simulink model "TST_Fans_trq"  (R2016b)
settings: Solver=FixedStepDiscrete  StartTime=0.0  StopTime=simTime  FixedStep=sampleTime  RelTol=1e-3
values from neighbouring files (symbols this model uses):
  testCase = 1    [initTST_Fans_trq_001.m]    (also in initTST_Fans_trq_002.m = 2)
libraries: simulink x7, UnitTest_Lib x4
settings Model: Creator=zhengjinyan  LastModifiedBy=zhengjinyan
settings DebuggingCC: SignalRangeChecking=error

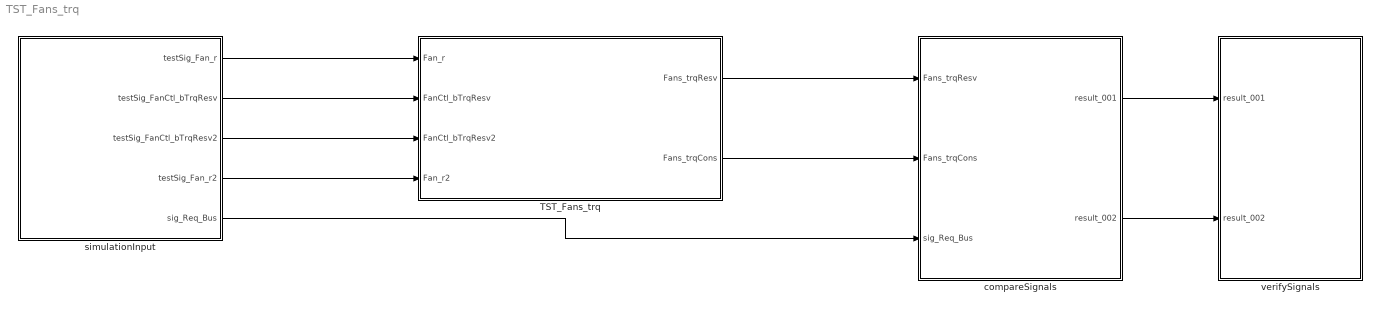
== system TST_Fans_trq ==
  TST_Fans_trq : Subsystem
  compareSignals : Subsystem
  simulationInput : Subsystem
  verifySignals : Subsystem
  wires:
  simulationInput/1(testSig_Fan_r) -> TST_Fans_trq/1(Fan_r)
  simulationInput/2(testSig_FanCtl_bTrqResv) -> TST_Fans_trq/2(FanCtl_bTrqResv)
  simulationInput/3(testSig_FanCtl_bTrqResv2) -> TST_Fans_trq/3(FanCtl_bTrqResv2)
  simulationInput/4(testSig_Fan_r2) -> TST_Fans_trq/4(Fan_r2)
  TST_Fans_trq/1(Fans_trqResv) -> compareSignals/1(Fans_trqResv)
  TST_Fans_trq/2(Fans_trqCons) -> compareSignals/2(Fans_trqCons)
  simulationInput/5(sig_Req_Bus) -> compareSignals/3(sig_Req_Bus)
  compareSignals/1(result_001) -> verifySignals/1(result_001)
  compareSignals/2(result_002) -> verifySignals/2(result_002)

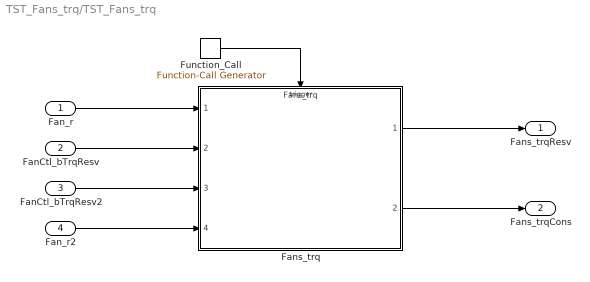
== system TST_Fans_trq/TST_Fans_trq ==
  Fan_r : Inport
  FanCtl_bTrqResv : Inport  Port=2
  FanCtl_bTrqResv2 : Inport  Port=3
  Fan_r2 : Inport  Port=4
  Fans_trq : ModelReference  ModelNameDialog=Fans_trq  SimulationMode=Normal  ModelReferenceVersion=1.16  TriggerPortName=function  TriggerPortTriggerType=function-call  TriggerPortStatesWhenEnabling=held
  Function_Call : simulink/Ports & Subsystems/Function-Call Generator  sample_time=sampleTime  numberOfIterations=1
  Fans_trqResv : Outport
  Fans_trqCons : Outport  Port=2
  wires:
  Function_Call/1 -> Fans_trq/Trigger
  Fan_r/1 -> Fans_trq/1
  FanCtl_bTrqResv/1 -> Fans_trq/2
  FanCtl_bTrqResv2/1 -> Fans_trq/3
  Fan_r2/1 -> Fans_trq/4
  Fans_trq/1 -> Fans_trqResv/1
  Fans_trq/2 -> Fans_trqCons/1

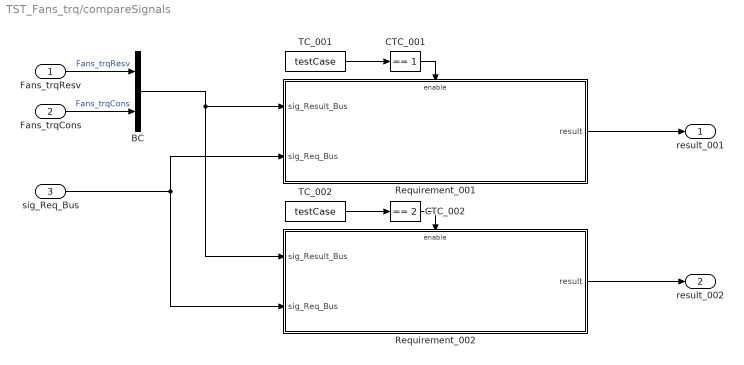
== system TST_Fans_trq/compareSignals ==
  Fans_trqResv : Inport
  Fans_trqCons : Inport  Port=2
  sig_Req_Bus : Inport  Port=3
  BC : BusCreator  Inputs=2
  CTC_001 : simulink/Logic and Bit Operations/Compare To Constant  relop===  const=1  OutDataTypeStr=boolean
  CTC_002 : simulink/Logic and Bit Operations/Compare To Constant  relop===  const=2  OutDataTypeStr=boolean
  Requirement_001 : Subsystem
  Requirement_002 : Subsystem
  TC_001 : Constant  Value=testCase
  TC_002 : Constant  Value=testCase
  result_001 : Outport
  result_002 : Outport  Port=2
  wires:
  Fans_trqResv/1 -> BC/1  "Fans_trqResv"
  Fans_trqCons/1 -> BC/2  "Fans_trqCons"
  TC_001/1 -> CTC_001/1
  CTC_001/1 -> Requirement_001/Enable
  sig_Req_Bus/1 -> Requirement_001/2(sig_Req_Bus), Requirement_002/2(sig_Req_Bus)
  BC/1 -> Requirement_001/1(sig_Result_Bus), Requirement_002/1(sig_Result_Bus)
  Requirement_001/1(result) -> result_001/1
  TC_002/1 -> CTC_002/1
  CTC_002/1 -> Requirement_002/Enable
  Requirement_002/1(result) -> result_002/1

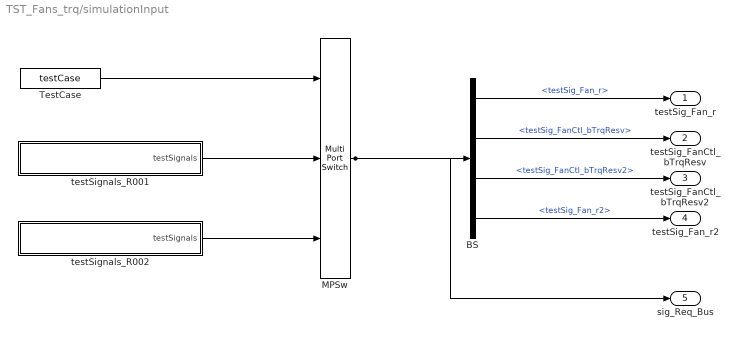
== system TST_Fans_trq/simulationInput ==
  BS : BusSelector  OutputSignals=testSig_Fan_r,testSig_FanCtl_bTrqResv,testSig_FanCtl_bTrqResv2,testSig_Fan_r2
  MPSw : MultiPortSwitch  Inputs=2  SaturateOnIntegerOverflow=on  InputSameDT=on
  TestCase : Constant  Value=testCase
  testSignals_R001 : Subsystem
  testSignals_R002 : Subsystem
  testSig_Fan_r : Outport
  testSig_FanCtl_bTrqResv : Outport  Port=2
  testSig_FanCtl_bTrqResv2 : Outport  Port=3
  testSig_Fan_r2 : Outport  Port=4
  sig_Req_Bus : Outport  Port=5
  wires:
  BS/1 -> testSig_Fan_r/1  "<testSig_Fan_r>"
  BS/2 -> testSig_FanCtl_bTrqResv/1  "<testSig_FanCtl_bTrqResv>"
  BS/3 -> testSig_FanCtl_bTrqResv2/1  "<testSig_FanCtl_bTrqResv2>"
  BS/4 -> testSig_Fan_r2/1  "<testSig_Fan_r2>"
  MPSw/1 -> BS/1, sig_Req_Bus/1
  TestCase/1 -> MPSw/1
  testSignals_R001/1(testSignals) -> MPSw/2
  testSignals_R002/1(testSignals) -> MPSw/3

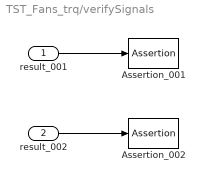
== system TST_Fans_trq/verifySignals ==
  result_001 : Inport
  result_002 : Inport  Port=2
  Assertion_001 : Assertion  Enabled=off
  Assertion_002 : Assertion  Enabled=off
  wires:
  result_001/1 -> Assertion_001/1
  result_002/1 -> Assertion_002/1

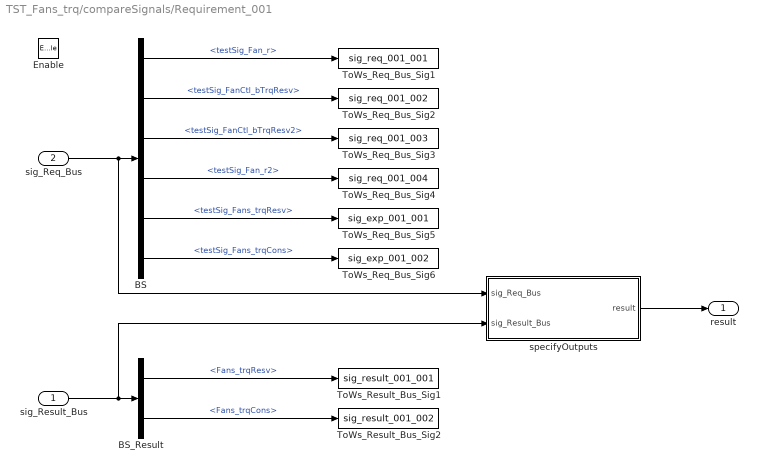
== system TST_Fans_trq/compareSignals/Requirement_001 ==
  sig_Result_Bus : Inport
  sig_Req_Bus : Inport  Port=2
  Enable : EnablePort
  BS : BusSelector  OutputSignals=testSig_Fan_r,testSig_FanCtl_bTrqResv,testSig_FanCtl_bTrqResv2,testSig_Fan_r2,testSig_Fans_trqResv,testSig_Fans_trqCons
  BS_Result : BusSelector  OutputSignals=Fans_trqResv,Fans_trqCons
  ToWs_Req_Bus_Sig1 : ToWorkspace  VariableName=sig_req_001_001  SaveFormat=Structure With Time
  ToWs_Req_Bus_Sig2 : ToWorkspace  VariableName=sig_req_001_002  SaveFormat=Structure With Time
  ToWs_Req_Bus_Sig3 : ToWorkspace  VariableName=sig_req_001_003  SaveFormat=Structure With Time
  ToWs_Req_Bus_Sig4 : ToWorkspace  VariableName=sig_req_001_004  SaveFormat=Structure With Time
  ToWs_Req_Bus_Sig5 : ToWorkspace  VariableName=sig_exp_001_001  SaveFormat=Structure With Time
  ToWs_Req_Bus_Sig6 : ToWorkspace  VariableName=sig_exp_001_002  SaveFormat=Structure With Time
  ToWs_Result_Bus_Sig1 : ToWorkspace  VariableName=sig_result_001_001  SaveFormat=Structure With Time
  ToWs_Result_Bus_Sig2 : ToWorkspace  VariableName=sig_result_001_002  SaveFormat=Structure With Time
  specifyOutputs : Subsystem
  result : Outport
  wires:
  sig_Req_Bus/1 -> BS/1, specifyOutputs/1(sig_Req_Bus)
  BS/1 -> ToWs_Req_Bus_Sig1/1  "<testSig_Fan_r>"
  BS/2 -> ToWs_Req_Bus_Sig2/1  "<testSig_FanCtl_bTrqResv>"
  BS/3 -> ToWs_Req_Bus_Sig3/1  "<testSig_FanCtl_bTrqResv2>"
  BS/4 -> ToWs_Req_Bus_Sig4/1  "<testSig_Fan_r2>"
  BS/5 -> ToWs_Req_Bus_Sig5/1  "<testSig_Fans_trqResv>"
  BS/6 -> ToWs_Req_Bus_Sig6/1  "<testSig_Fans_trqCons>"
  sig_Result_Bus/1 -> BS_Result/1, specifyOutputs/2(sig_Result_Bus)
  BS_Result/1 -> ToWs_Result_Bus_Sig1/1  "<Fans_trqResv>"
  BS_Result/2 -> ToWs_Result_Bus_Sig2/1  "<Fans_trqCons>"
  specifyOutputs/1(result) -> result/1

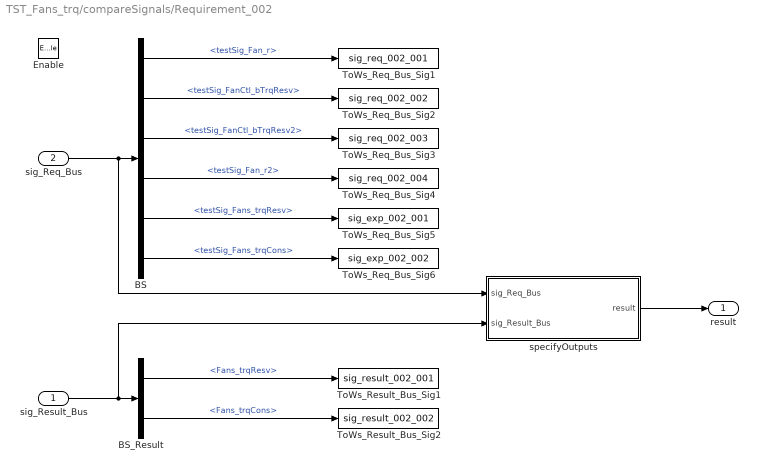
== system TST_Fans_trq/compareSignals/Requirement_002 ==
  sig_Result_Bus : Inport
  sig_Req_Bus : Inport  Port=2
  Enable : EnablePort
  BS : BusSelector  OutputSignals=testSig_Fan_r,testSig_FanCtl_bTrqResv,testSig_FanCtl_bTrqResv2,testSig_Fan_r2,testSig_Fans_trqResv,testSig_Fans_trqCons
  BS_Result : BusSelector  OutputSignals=Fans_trqResv,Fans_trqCons
  ToWs_Req_Bus_Sig1 : ToWorkspace  VariableName=sig_req_002_001  SaveFormat=Structure With Time
  ToWs_Req_Bus_Sig2 : ToWorkspace  VariableName=sig_req_002_002  SaveFormat=Structure With Time
  ToWs_Req_Bus_Sig3 : ToWorkspace  VariableName=sig_req_002_003  SaveFormat=Structure With Time
  ToWs_Req_Bus_Sig4 : ToWorkspace  VariableName=sig_req_002_004  SaveFormat=Structure With Time
  ToWs_Req_Bus_Sig5 : ToWorkspace  VariableName=sig_exp_002_001  SaveFormat=Structure With Time
  ToWs_Req_Bus_Sig6 : ToWorkspace  VariableName=sig_exp_002_002  SaveFormat=Structure With Time
  ToWs_Result_Bus_Sig1 : ToWorkspace  VariableName=sig_result_002_001  SaveFormat=Structure With Time
  ToWs_Result_Bus_Sig2 : ToWorkspace  VariableName=sig_result_002_002  SaveFormat=Structure With Time
  specifyOutputs : Subsystem
  result : Outport
  wires:
  sig_Req_Bus/1 -> BS/1, specifyOutputs/1(sig_Req_Bus)
  BS/1 -> ToWs_Req_Bus_Sig1/1  "<testSig_Fan_r>"
  BS/2 -> ToWs_Req_Bus_Sig2/1  "<testSig_FanCtl_bTrqResv>"
  BS/3 -> ToWs_Req_Bus_Sig3/1  "<testSig_FanCtl_bTrqResv2>"
  BS/4 -> ToWs_Req_Bus_Sig4/1  "<testSig_Fan_r2>"
  BS/5 -> ToWs_Req_Bus_Sig5/1  "<testSig_Fans_trqResv>"
  BS/6 -> ToWs_Req_Bus_Sig6/1  "<testSig_Fans_trqCons>"
  sig_Result_Bus/1 -> BS_Result/1, specifyOutputs/2(sig_Result_Bus)
  BS_Result/1 -> ToWs_Result_Bus_Sig1/1  "<Fans_trqResv>"
  BS_Result/2 -> ToWs_Result_Bus_Sig2/1  "<Fans_trqCons>"
  specifyOutputs/1(result) -> result/1

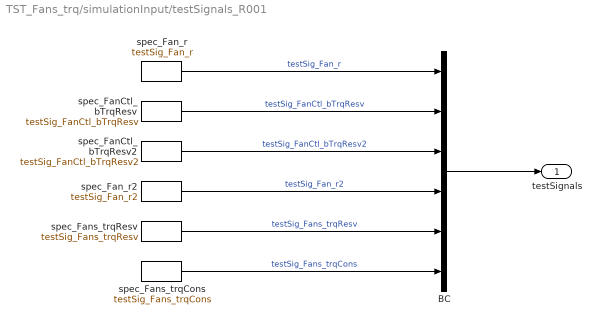
== system TST_Fans_trq/simulationInput/testSignals_R001 ==
  BC : BusCreator  Inputs=6
  spec_FanCtl_bTrqResv : FromWorkspace  VariableName=testSig_FanCtl_bTrqResv  Interpolate=off  OutputAfterFinalValue=Holding final value
  spec_FanCtl_bTrqResv2 : FromWorkspace  VariableName=testSig_FanCtl_bTrqResv2  Interpolate=off  OutputAfterFinalValue=Holding final value
  spec_Fan_r : FromWorkspace  VariableName=testSig_Fan_r  Interpolate=off  OutputAfterFinalValue=Holding final value
  spec_Fan_r2 : FromWorkspace  VariableName=testSig_Fan_r2  Interpolate=off  OutputAfterFinalValue=Holding final value
  spec_Fans_trqCons : FromWorkspace  VariableName=testSig_Fans_trqCons  Interpolate=off  OutputAfterFinalValue=Holding final value
  spec_Fans_trqResv : FromWorkspace  VariableName=testSig_Fans_trqResv  Interpolate=off  OutputAfterFinalValue=Holding final value
  testSignals : Outport
  wires:
  BC/1 -> testSignals/1
  spec_Fan_r/1 -> BC/1  "testSig_Fan_r"
  spec_FanCtl_bTrqResv/1 -> BC/2  "testSig_FanCtl_bTrqResv"
  spec_FanCtl_bTrqResv2/1 -> BC/3  "testSig_FanCtl_bTrqResv2"
  spec_Fan_r2/1 -> BC/4  "testSig_Fan_r2"
  spec_Fans_trqResv/1 -> BC/5  "testSig_Fans_trqResv"
  spec_Fans_trqCons/1 -> BC/6  "testSig_Fans_trqCons"

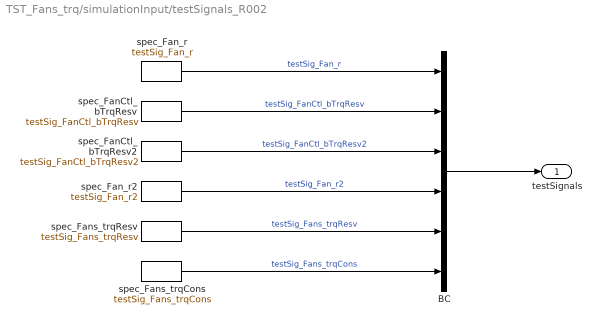
== system TST_Fans_trq/simulationInput/testSignals_R002 ==
  BC : BusCreator  Inputs=6
  spec_FanCtl_bTrqResv : FromWorkspace  VariableName=testSig_FanCtl_bTrqResv  Interpolate=off  OutputAfterFinalValue=Holding final value
  spec_FanCtl_bTrqResv2 : FromWorkspace  VariableName=testSig_FanCtl_bTrqResv2  Interpolate=off  OutputAfterFinalValue=Holding final value
  spec_Fan_r : FromWorkspace  VariableName=testSig_Fan_r  Interpolate=off  OutputAfterFinalValue=Holding final value
  spec_Fan_r2 : FromWorkspace  VariableName=testSig_Fan_r2  Interpolate=off  OutputAfterFinalValue=Holding final value
  spec_Fans_trqCons : FromWorkspace  VariableName=testSig_Fans_trqCons  Interpolate=off  OutputAfterFinalValue=Holding final value
  spec_Fans_trqResv : FromWorkspace  VariableName=testSig_Fans_trqResv  Interpolate=off  OutputAfterFinalValue=Holding final value
  testSignals : Outport
  wires:
  BC/1 -> testSignals/1
  spec_Fan_r/1 -> BC/1  "testSig_Fan_r"
  spec_FanCtl_bTrqResv/1 -> BC/2  "testSig_FanCtl_bTrqResv"
  spec_FanCtl_bTrqResv2/1 -> BC/3  "testSig_FanCtl_bTrqResv2"
  spec_Fan_r2/1 -> BC/4  "testSig_Fan_r2"
  spec_Fans_trqResv/1 -> BC/5  "testSig_Fans_trqResv"
  spec_Fans_trqCons/1 -> BC/6  "testSig_Fans_trqCons"

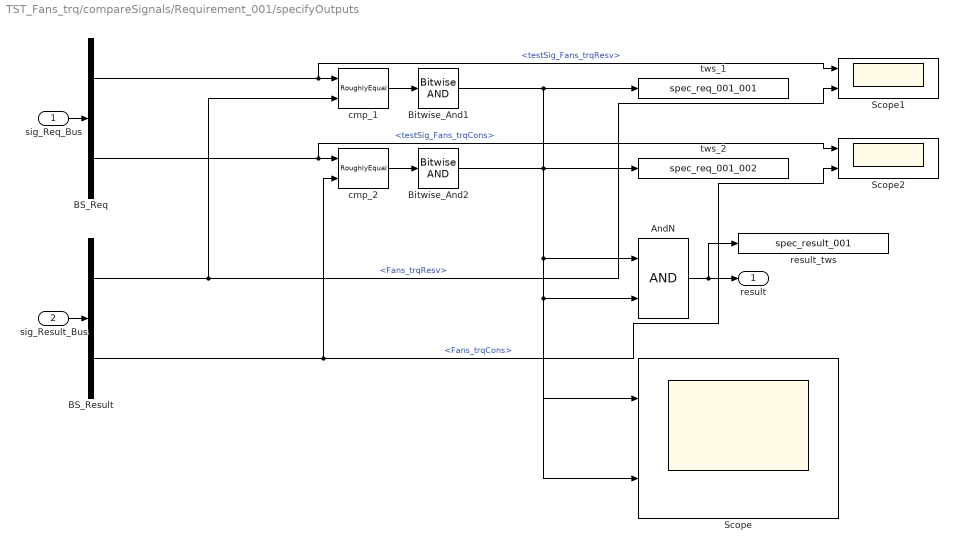
== system TST_Fans_trq/compareSignals/Requirement_001/specifyOutputs ==
  sig_Req_Bus : Inport
  sig_Result_Bus : Inport  Port=2
  AndN : Logic
  BS_Req : BusSelector  OutputSignals=testSig_Fans_trqResv,testSig_Fans_trqCons
  BS_Result : BusSelector  OutputSignals=Fans_trqResv,Fans_trqCons
  Bitwise_And1 : simulink/Logic and Bit Operations/Bitwise Operator  logicop=AND  UseBitMask=off  BitMask=bin2dec('11011001')  BitMaskRealWorld=Stored Integer
  Bitwise_And2 : simulink/Logic and Bit Operations/Bitwise Operator  logicop=AND  UseBitMask=off  BitMask=bin2dec('11011001')  BitMaskRealWorld=Stored Integer
  Scope : Scope  NumInputPorts=2
  Scope1 : Scope  NumInputPorts=2
  Scope2 : Scope  NumInputPorts=2
  cmp_1 : UnitTest_Lib/RoughlyEqual  slope=2
  cmp_2 : UnitTest_Lib/RoughlyEqual  slope=2
  result_tws : ToWorkspace  VariableName=spec_result_001
  tws_1 : ToWorkspace  VariableName=spec_req_001_001
  tws_2 : ToWorkspace  VariableName=spec_req_001_002
  result : Outport
  wires:
  sig_Req_Bus/1 -> BS_Req/1
  sig_Result_Bus/1 -> BS_Result/1
  AndN/1 -> result/1, result_tws/1
  BS_Req/1 -> cmp_1/1, Scope1/1  "<testSig_Fans_trqResv>"
  BS_Result/1 -> cmp_1/2, Scope1/2  "<Fans_trqResv>"
  cmp_1/1 -> Bitwise_And1/1
  Bitwise_And1/1 -> AndN/1, Scope/1, tws_1/1
  BS_Req/2 -> cmp_2/1, Scope2/1  "<testSig_Fans_trqCons>"
  BS_Result/2 -> cmp_2/2, Scope2/2  "<Fans_trqCons>"
  cmp_2/1 -> Bitwise_And2/1
  Bitwise_And2/1 -> AndN/2, Scope/2, tws_2/1

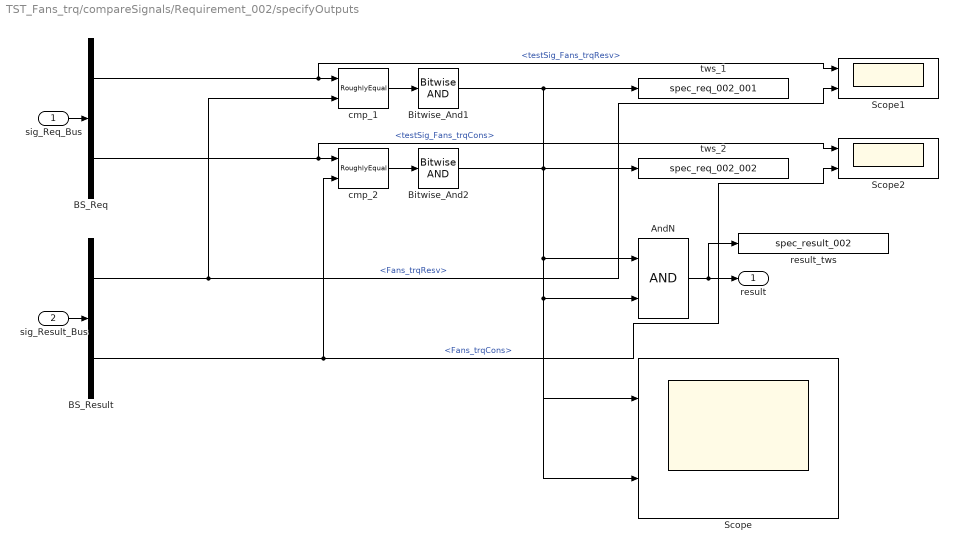
== system TST_Fans_trq/compareSignals/Requirement_002/specifyOutputs ==
  sig_Req_Bus : Inport
  sig_Result_Bus : Inport  Port=2
  AndN : Logic
  BS_Req : BusSelector  OutputSignals=testSig_Fans_trqResv,testSig_Fans_trqCons
  BS_Result : BusSelector  OutputSignals=Fans_trqResv,Fans_trqCons
  Bitwise_And1 : simulink/Logic and Bit Operations/Bitwise Operator  logicop=AND  UseBitMask=off  BitMask=bin2dec('11011001')  BitMaskRealWorld=Stored Integer
  Bitwise_And2 : simulink/Logic and Bit Operations/Bitwise Operator  logicop=AND  UseBitMask=off  BitMask=bin2dec('11011001')  BitMaskRealWorld=Stored Integer
  Scope : Scope  NumInputPorts=2
  Scope1 : Scope  NumInputPorts=2
  Scope2 : Scope  NumInputPorts=2
  cmp_1 : UnitTest_Lib/RoughlyEqual  slope=2
  cmp_2 : UnitTest_Lib/RoughlyEqual  slope=2
  result_tws : ToWorkspace  VariableName=spec_result_002
  tws_1 : ToWorkspace  VariableName=spec_req_002_001
  tws_2 : ToWorkspace  VariableName=spec_req_002_002
  result : Outport
  wires:
  sig_Req_Bus/1 -> BS_Req/1
  sig_Result_Bus/1 -> BS_Result/1
  AndN/1 -> result/1, result_tws/1
  BS_Req/1 -> cmp_1/1, Scope1/1  "<testSig_Fans_trqResv>"
  BS_Result/1 -> cmp_1/2, Scope1/2  "<Fans_trqResv>"
  cmp_1/1 -> Bitwise_And1/1
  Bitwise_And1/1 -> AndN/1, Scope/1, tws_1/1
  BS_Req/2 -> cmp_2/1, Scope2/1  "<testSig_Fans_trqCons>"
  BS_Result/2 -> cmp_2/2, Scope2/2  "<Fans_trqCons>"
  cmp_2/1 -> Bitwise_And2/1
  Bitwise_And2/1 -> AndN/2, Scope/2, tws_2/1
